simulink model "M_QAM"  (R2025b)
settings: Solver=VariableStepAuto  StartTime=0.0  StopTime=10.0  RelTol=1e-3
undefined symbols (not defined in the file or in its folder): qammod
libraries: commdigbbndam3 x2, commsink2 x2, simulink x2, commchan3 x1, commrandsrc3 x1
settings Model: Creator=namit  LastModifiedBy=namit

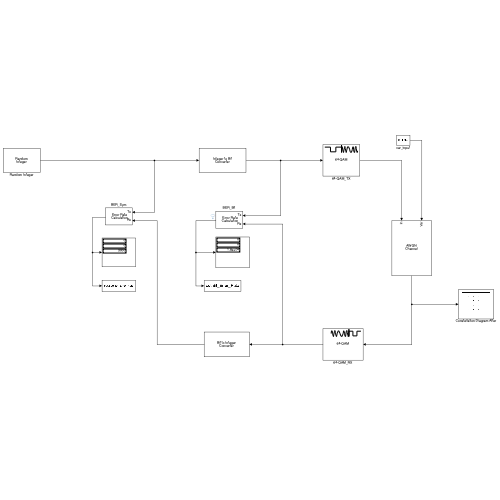
[thumbnail: Simulink's stored preview of the top-level diagram]
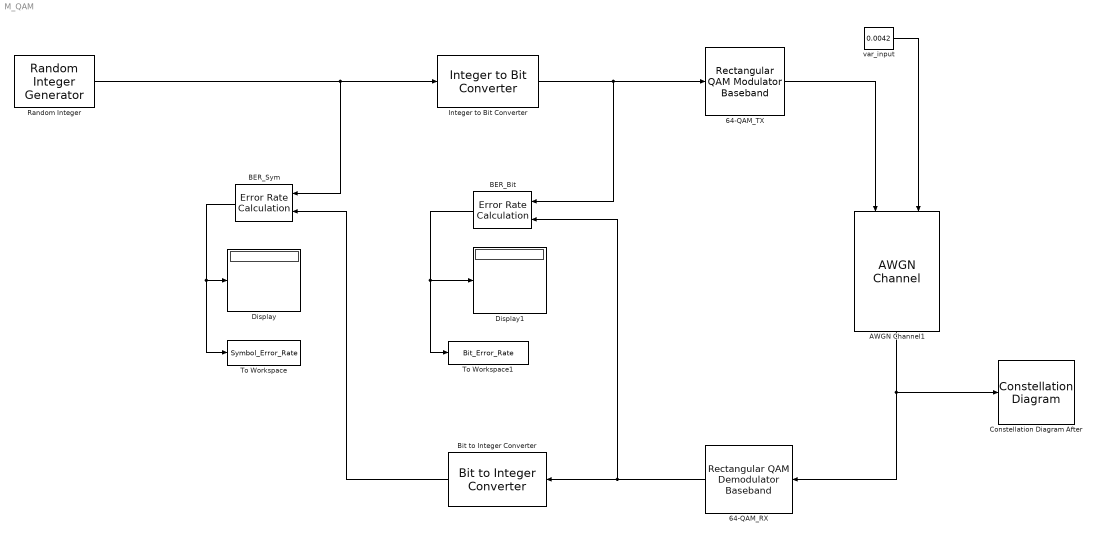
== system M_QAM ==
  64-QAM_RX : commdigbbndam3/Rectangular QAM Demodulator Baseband  M=64  OutType=Bit  DecType=Hard decision  VarSource=Dialog  Variance=1  Dec=Gray  Mapping=[0:15]  PowType=Min. distance between symbols  MinDist=2  AvgPow=1  PeakPow=1  Ph=0  outDtype1=Inherit via internal rule  outDtype2=Inherit via internal rule  derotateFactorWordLen=16  derotateFactorDataTypeStr=Inherit: Same word length as input  derotateFactorLastDataTypeStr=Inherit: Same word length as input  denormFactorWordLen=16  denormFactorDataTypeStr=Inherit: Same word length as input  denormFactorLastDataTypeStr=Inherit: Same word length as input  prodOutWordLen=32  prodOutOverflowMode=Wrap  prodOutRoundingMode=Floor  prodOutOvFlMode=off  prodOutOvFlModeLastStrValue=off  sumWordLen=32
  64-QAM_TX : commdigbbndam3/Rectangular QAM Modulator Baseband  M=64  InType=Bit  Enc=Gray  Mapping=[0:15]  PowType=Min. distance between symbols  MinDist=2  AvgPow=1  PeakPow=1  Ph=0  outDtype=double  outWordLen=16  outUDDataType=sfix(16)  outFracLenMode=Best precision  outFracLen=15  outDataTypeStr=double  outLastDataTypeStr=double
  AWGN Channel1 : commchan3/AWGN Channel  LegacyMode=off  NoiseMethod=Variance  noiseMode="Signal to noise ratio  (SNR)"  EbNo=10  EsNo=10  SNR=10  BitsPerSymbol=1  SignalPower=1  SpecifySymbolPeriod=off  SamplesPerSymbol=1  SymbolPeriod=1  VarianceSource=Input port  Variance=1  RandomStream=Global stream  Seed=67  SimulateUsing=Interpreted execution
  BER_Bit : commsink2/Error Rate Calculation  N=0  st_delay=0  cp_mode=Entire frame  subframe=[]  PMode=Port  WsName=ErrorVec  RsMode2=off  stop=off  numErr=100  maxBits=1e6
  BER_Sym : commsink2/Error Rate Calculation  N=0  st_delay=0  cp_mode=Entire frame  subframe=[]  PMode=Port  WsName=ErrorVec  RsMode2=off  stop=off  numErr=100  maxBits=1e6
  Bit to Integer Converter : simulink/Logic and Bit Operations/Bit to Integer Converter  nbits=6  bitOrder=MSB first  signedOutputValues=Unsigned  outDtype=Inherit via internal rule  outDtypeSigned=Inherit via internal rule
      settings: LibrarySourceBlock=|
      | commutil2/Bit to Integer
      | Converter
  Constellation Diagram After : ConstellationDiagram  WindowPosition=[1.000000,1.000000,1470.000000,923.000000,]  Visible=on  ScopeFrameLocation=window  ReferenceConstellation=qammod(0:63, 64)
  Display : Display
  Display1 : Display
  Integer to Bit Converter : simulink/Logic and Bit Operations/Integer to Bit Converter  nbits=6  signedInputValues=Unsigned  bitOrder=MSB first  outDtype=Inherit via internal rule
      settings: LibrarySourceBlock=|
      | commutil2/Integer to Bit
      | Converter
  Random Integer : commrandsrc3/Random Integer Generator  SetSize=64  SeedSource=Auto  Seed=0  SampleTime=1  SamplesPerFrame=3000  OutputDataType=double  SimulateUsing=Interpreted execution
  To Workspace : ToWorkspace  VariableName=Symbol_Error_Rate  SampleTime=-1
  To Workspace1 : ToWorkspace  VariableName=Bit_Error_Rate  SampleTime=-1
  var_input : Constant  Value=0.0042
  wires:
  Random Integer/1 -> Integer to Bit Converter/1, BER_Sym/1
  Integer to Bit Converter/1 -> 64-QAM_TX/1, BER_Bit/1
  var_input/1 -> AWGN Channel1/2
  64-QAM_TX/1 -> AWGN Channel1/1
  AWGN Channel1/1 -> 64-QAM_RX/1, Constellation Diagram After/1
  64-QAM_RX/1 -> BER_Bit/2, Bit to Integer Converter/1
  BER_Bit/1 -> To Workspace1/1, Display1/1
  BER_Sym/1 -> To Workspace/1, Display/1
  Bit to Integer Converter/1 -> BER_Sym/2
